simulink model "cubli_model"  (R2017a)
settings: Solver=VariableStepAuto  StartTime=0.0  StopTime=10.0  RelTol=1e-3
values from neighbouring files (symbols this model uses):
  Km = 25.1e-3    (= 0.0251)    [parameters.m]
undefined symbols (not defined in the file or in its folder): thb0, thb_d0, thw0, thw_d0, Um
settings Model: Creator=gdiazh  LastModifiedBy=gdiazh

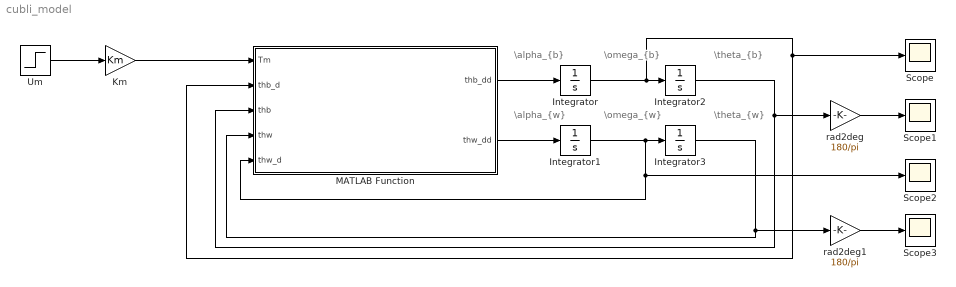
== system cubli_model ==
  note: \alpha_{b}
  note: \alpha_{w}
  note: \omega_{b}
  note: \omega_{w}
  note: \theta_{b}
  note: \theta_{w}
  Integrator : Integrator  InitialCondition=thb_d0
  Integrator1 : Integrator  InitialCondition=thw_d0
  Integrator2 : Integrator  InitialCondition=thb0
  Integrator3 : Integrator  InitialCondition=thw0
  Km : Gain  Gain=Km
  MATLAB Function : MATLAB Function  TreatAsAtomicUnit=on
  Scope{,1..3} (4 alike) : Scope
  Um : Step  After=Um  SampleTime=0
  rad2deg : Gain  Gain=180/pi
  rad2deg1 : Gain  Gain=180/pi
  wires:
  Integrator/1 -> Scope/1, MATLAB Function/2(thb_d), Integrator2/1
  MATLAB Function/1(thb_dd) -> Integrator/1
  MATLAB Function/2(thw_dd) -> Integrator1/1
  Integrator1/1 -> Scope2/1, MATLAB Function/5(thw_d), Integrator3/1
  Integrator3/1 -> MATLAB Function/4(thw), rad2deg1/1
  Integrator2/1 -> rad2deg/1, MATLAB Function/3(thb)
  Um/1 -> Km/1
  Km/1 -> MATLAB Function/1(Tm)
  rad2deg/1 -> Scope1/1
  rad2deg1/1 -> Scope3/1

== matlab function cubli_model/MATLAB Function ==
  data: Tm input; thb_d input; thb input; thb_dd output; thw input; thw_d input; thw_dd output
function [thb_dd, thw_dd] = inverted_pendulum(Tm, thb_d, thb, thw, thw_d)
    
    % Model parameters
    l = 0.085; 		%[m]
    lb = 0.075;		%[m]
    mb = 0.419;		%[Kg]
    mw = 0.204;		%[Kg]
    Ib = 3.34e-3;	%[Kgm2]
    Iw = 0.57e-3;	%[Kgm2]
    Cb = 1.02e-3;	%[Kgm2s-1]
    Cw = 0.05e-3;	%[Kgm2s-1]
    g = 9.8;		%[m/s2]
    Km = 25.1e-3;	%[NmA-1]

    thb_dd = ((mb*lb+mw*l)*g*sin(thb)-Tm-Cb*thb_d+Cw*thw_d)/(Ib+mw*l^2);
    thw_dd = ((Ib+Iw+mw*l^2)*(Tm-Cw*thw_d))/(Iw*(Ib+mw*l^2)) - ((mb*lb+mw*l)*g*sin(thb)-Cb*thb_d)/(Ib+mw*l^2);
end
